simulink model "bldc_lab"  (R2021b)
settings: Solver=ode15s  StartTime=0.0  StopTime=2  FixedStep=0.0000005  MaxStep=0.000001  RelTol=1e-3
undefined symbols (not defined in the file): Ion, Lithium
libraries: spsIGBTDiodeLib x8, slpidlib x2, spsVoltageMeasurementLib x2, spsSeriesRLCBranchLib x2, spsBatteryLib x1, spsCurrentMeasurementLib x1, spsDCVoltageSourceLib x1, spsPermanentMagnetSynchronousMachineLib x1, spsIdealSwitchLib x1, spsPWMGeneratorDCDCLib x1, spspowerguiLib x1
settings Model: Creator=borutzki  LastModifiedBy=borutzki
settings SolverCC: ZeroCrossAlgorithm=Adaptive
settings DebuggingCC: IgnoredZcDiagnostic=none

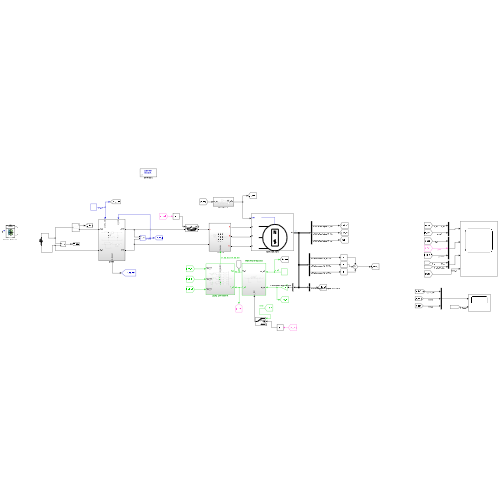
[thumbnail: Simulink's stored preview of the top-level diagram]
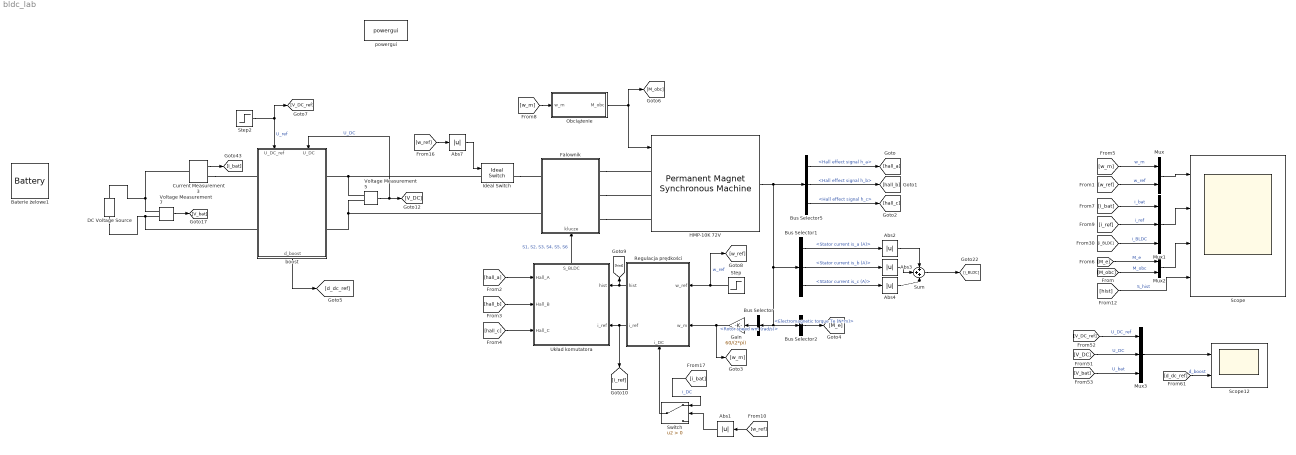
== system bldc_lab ==
  Abs{1..4,7} (5 alike) : Abs
  Baterie żelowe1 : spsBatteryLib/Battery  BatType=Lithium-Ion  ShowTempParam=off  ThermalPreset=no  ShowAgeParam=off  NomV=36  NomQ=5  SOC=100  Batt_Tr=30  PresetModel=on  MaxQ=5  MinV=27  FullV=41.9035  Dis_rate=2.1739  R=0.072  Normal_OP=4.5217  expZone="[38.8939     0.245652]"  current=[6.5 13 32.5]  Units=Time  Tci=20  NomT=20  T2=-30  MaxQ2=4.8  FullV2=7.1  Normal_OP2=5.655  expZone2="[6.58           1]"  Rca=0.6  ti=2000  Dp=0  Neq0=0  Tsim=1e6  Ta1=25  Qeol=5.4*0.9  Reol=0.013333*1.2  Char_age=[2.3478, 3]  Dis_age=[2.3478, 10]  N1=1500  N2=10500  N3=1000  N4=1400  Ta2=45  N5=950
  Bus Selector : BusSelector  OutputSignals=Rotor speed wm (rad/s)
  Bus Selector1 : BusSelector  OutputSignals=Stator current is_a (A),Stator current is_b (A),Stator current is_c (A)
  Bus Selector2 : BusSelector  OutputSignals=Electromagnetic torque Te (N*m)
  Bus Selector5 : BusSelector  OutputSignals=Hall effect signal h_a,Hall effect signal h_b,Hall effect signal h_c
  Current Measurement3 : spsCurrentMeasurementLib/Current Measurement  PhasorSimulation=off  OutputType=Complex  PSBequivalent=0
  DC Voltage Source : spsDCVoltageSourceLib/DC Voltage Source  Amplitude=36  Measurements=None
  Falownik : Subsystem
      settings: PortSchema="{\"entries\":[{\"content\":{\"sides\":[{\"content\":{\"connectorIds\":[\"LConn1\",\"LConn2\"]},\"type\":\"ConnectorPlacement.EquallySpacedRectSide\",\"uuid\":\"21967f67-7ecc-4de4-91fd-b00cf07b6fbf\"},{\"content\":{\"connectorIds\":[\"RConn1\",\"RConn2\",\"RConn3\"],\"side\":\"RIGHT\"},\"type\":\"ConnectorPlacement.EquallySpacedRectSide\",\"uuid\":\"18bc580d-fbaa-4fc1-af99-2ad48ced499f\"},{\"content\":{\"connectorIds\":[],\"side\":\"TOP\"},\"type\":\"ConnectorPlacement.EquallySpacedRectSide\",\"uuid\":\"29f4965a-54f7-4925-8e4b-dbb7ca0827f0\"},{\"content\":{\"connectorIds\":[\"In1\"],\"side\":\"BOTTOM\"},\"type\":\"ConnectorPlacement.EquallySpacedRectSide\",\"uuid\":\"6d9bc2af-b4ca-4c5d-94c1-33ab2980993d\"}]},\"type\":\"ConnectorPlacement.EquallySpacedConnector\",\"uuid\":\"e72db418-b731-4ad1-a158-dfab229f0014\"}],\"packageUris\":[\"http://schema.mathworks.com/mf0/Connector/R2020b\"],\"version\":\"1.0\"}"
  Gain : Gain  Gain=60/(2*pi)
  HMP-10K 72V : spsPermanentMagnetSynchronousMachineLib/Permanent Magnet Synchronous Machine  NbPhases=3  FluxDistribution=Trapezoidal  RotorType=Round  MechanicalLoad=Torque Tm  PresetModel=No  ShowDetailedParameters=on  MeasurementBus=off  Resistance=0.00265  Inductance=5.2e-08  dqInductances=[8.5e-3,8.5e-3]  La=0.000835  MachineConstant=Flux linkage established by magnets (V.s)  Flux=0.0198529  VoltageCst=16.6319  TorqueCst=0.15882  Flat=120  Mechanical=[0.000621417 0 4]  PolePairs=4  InitialConditions=[0,0, 0,0]  InitialConditions5ph=[0 0 0 0 0 0]  RefAngle=90 degrees behind phase A axis (modified Park)  IterativeDiscreteModel=Trapezoidal non iterative  TsBlock=-1  TsPowergui=0
  Ideal Switch : spsIdealSwitchLib/Ideal Switch  Ron=0.001  Lon=0  IC=0  Rs=10e8  Cs=inf  Measurements=on
  Mux : Mux  Inputs=2
  Mux1 : Mux  Inputs=3
  Mux2 : Mux  Inputs=2
  Mux3 : Mux  Inputs=3
  Obciążenie : Subsystem
  Regulacja prędkości : Subsystem
      settings: PortSchema="{\"entries\":[{\"content\":{\"sides\":[{\"content\":{\"connectorIds\":[\"In1\",\"In2\"]},\"type\":\"ConnectorPlacement.EquallySpacedRectSide\",\"uuid\":\"eb00a588-3794-4546-a1d2-9e4e9993d45f\"},{\"content\":{\"connectorIds\":[\"Out1\",\"Out2\"],\"side\":\"RIGHT\"},\"type\":\"ConnectorPlacement.EquallySpacedRectSide\",\"uuid\":\"a8ca2baf-3f9d-4e61-8f3e-3dda34de3f56\"},{\"content\":{\"connectorIds\":[],\"side\":\"TOP\"},\"type\":\"ConnectorPlacement.EquallySpacedRectSide\",\"uuid\":\"d8951c20-e465-4982-8368-20723ce9e6f9\"},{\"content\":{\"connectorIds\":[\"In3\"],\"side\":\"BOTTOM\"},\"type\":\"ConnectorPlacement.EquallySpacedRectSide\",\"uuid\":\"c6264e01-0c9f-421a-afb1-88d153170c6d\"}]},\"type\":\"ConnectorPlacement.EquallySpacedConnector\",\"uuid\":\"1286fe2f-7144-491a-9d4a-5774b4a98f05\"}],\"packageUris\":[\"http://schema.mathworks.com/mf0/Connector/R2020b\"],\"version\":\"1.0\"}"
  Scope : Scope  NumInputPorts=4
  Scope12 : Scope  NumInputPorts=2
  Step : Step  Time=0.5  After=500  SampleTime=0
  Step2 : Step  Time=0.2  After=72  SampleTime=0
  Sum : Sum  Inputs=+++
  Switch : Switch  Criteria=u2 > Threshold
  Układ komutatora : Subsystem
      settings: PortSchema="{\"entries\":[{\"content\":{\"sides\":[{\"content\":{\"connectorIds\":[\"In1\",\"In2\",\"In3\"]},\"type\":\"ConnectorPlacement.EquallySpacedRectSide\",\"uuid\":\"5145dd98-6096-41fa-a175-964c14778fb3\"},{\"content\":{\"connectorIds\":[\"In4\",\"In5\"],\"side\":\"RIGHT\"},\"type\":\"ConnectorPlacement.EquallySpacedRectSide\",\"uuid\":\"5175d556-6ef4-4a11-8093-81f2c4398356\"},{\"content\":{\"connectorIds\":[\"Out1\"],\"side\":\"TOP\"},\"type\":\"ConnectorPlacement.EquallySpacedRectSide\",\"uuid\":\"b6e9d80c-0e29-4a5b-b8c8-415c389c051e\"},{\"content\":{\"connectorIds\":[],\"side\":\"BOTTOM\"},\"type\":\"ConnectorPlacement.EquallySpacedRectSide\",\"uuid\":\"62976cb5-df0e-4349-b1ac-ce6e1718b9a9\"}]},\"type\":\"ConnectorPlacement.EquallySpacedConnector\",\"uuid\":\"8e04dc5d-fea8-4475-a1f4-09d0ee33eb3d\"}],\"packageUris\":[\"http://schema.mathworks.com/mf0/Connector/R2020b\"],\"version\":\"1.0\"}"
  Voltage Measurement5 : spsVoltageMeasurementLib/Voltage Measurement  PhasorSimulation=off  OutputType=Complex  PSBequivalent=0
  Voltage Measurement7 : spsVoltageMeasurementLib/Voltage Measurement  PhasorSimulation=off  OutputType=Complex  PSBequivalent=0
  boost : Subsystem
      settings: PortSchema="{\"entries\":[{\"content\":{\"sides\":[{\"content\":{\"connectorIds\":[\"LConn1\",\"LConn2\"]},\"type\":\"ConnectorPlacement.EquallySpacedRectSide\",\"uuid\":\"4c742702-5063-4be9-90fa-f2ecfe683f39\"},{\"content\":{\"connectorIds\":[\"RConn1\",\"RConn2\"],\"side\":\"RIGHT\"},\"type\":\"ConnectorPlacement.EquallySpacedRectSide\",\"uuid\":\"6758a030-dee0-40f5-ab65-dbe6d9640e0b\"},{\"content\":{\"connectorIds\":[\"In1\",\"In2\"],\"side\":\"TOP\"},\"type\":\"ConnectorPlacement.EquallySpacedRectSide\",\"uuid\":\"71135b2c-1a2a-4dc9-8a7c-02ce7c2ac3cd\"},{\"content\":{\"connectorIds\":[\"Out1\"],\"side\":\"BOTTOM\"},\"type\":\"ConnectorPlacement.EquallySpacedRectSide\",\"uuid\":\"cd62799b-22c9-45d9-9a7c-0387e77ecd9b\"}]},\"type\":\"ConnectorPlacement.EquallySpacedConnector\",\"uuid\":\"113fdbd2-88dc-4715-bf53-b53f7b5d75de\"}],\"packageUris\":[\"http://schema.mathworks.com/mf0/Connector/R2020b\"],\"version\":\"1.0\"}"
  powergui : spspowerguiLib/powergui  Priority=1  SimulationMode=Discrete  SampleTime=0.000005  frequency=60  Iterations=50  frequencyindice=0  Pbase=100e6  ErrMax=1e-4  UnitsV=kV  UnitsW=MW  buscounter=0  FunctionMessages=off  echomessages=off  EnableUseOfTLC=off  CurrentSourceSwitches=off  DisableSnubberDevices=off  DisableRonSwitches=off  DisableVfSwitches=off  DisplayEquations=off  AutomaticDiscreteSolvers=on  SolverType=Tustin/Backward Euler (TBE)  Interpol=off  ExternalGateDelay=off  methode=off  Ts=100  x0status=blocks  SPID=on  SwTol=0  HookPort=off  NonlinearTolerance=1e-4  nMaxIteration=100  ContinueOnMaxIteration=off  RestoreLinks=warning  ResistiveCurrentMeasurement=off  Frange=[0:2:500]  Ylog=off  Xlog=on  ShowGrid=off  save=off  variable=ZData  structure=0  ZoomFFT=off  StartTime=0.0  cycles=1  DisplayStyle=1  fundamental=60  FreqAxis=off  MaxFrequency=1000  frequencyindicesteady=1  RmsSteady=1  display=off
  wires:
  Bus Selector5/1 -> [hall_a]  "<Hall effect signal h_a>"
  Bus Selector5/2 -> [hall_b]  "<Hall effect signal h_b>"
  Bus Selector5/3 -> [hall_c]  "<Hall effect signal h_c>"
  [i_bat] -> Mux1/1  "i_bat"
  Voltage Measurement5/1 -> boost/2(U_DC), [V_DC]  "U_DC"
  Voltage Measurement7/1 -> [V_bat]
  Current Measurement3/1 -> [i_bat]
  [d_dc_ref] -> Scope12/2  "d_boost"
  [V_bat] -> Mux3/3  "U_bat"
  Mux3/1 -> Scope12/1
  [V_DC_ref] -> Mux3/1  "U_DC_ref"
  [V_DC] -> Mux3/2  "U_DC"
  [w_m] -> Mux/1  "w_m"
  [w_ref] -> Mux/2  "w_ref"
  Mux/1 -> Scope/1
  [i_ref] -> Mux1/2  "i_ref"
  Mux1/1 -> Scope/2
  [hist] -> Scope/4  "S_hist"
  Bus Selector1/3 -> Abs4/1  "<Stator current is_c (A)>"
  Bus Selector1/2 -> Abs3/1  "<Stator current is_b (A)>"
  Bus Selector1/1 -> Abs2/1  "<Stator current is_a (A)>"
  Abs2/1 -> Sum/1
  Abs3/1 -> Sum/2
  Abs4/1 -> Sum/3
  Sum/1 -> [i_BLDC]
  [i_BLDC] -> Mux1/3  "i_BLDC"
  [w_ref] -> Abs7/1
  Abs7/1 -> Ideal Switch/1
  Step2/1 -> boost/1(U_DC_ref), [V_DC_ref]  "U_ref"
  boost/1(d_boost) -> [d_dc_ref]
  [w_m] -> Obciążenie/1(w_m)
  [hall_a] -> Układ komutatora/1(Hall_A)
  [hall_b] -> Układ komutatora/2(Hall_B)
  [hall_c] -> Układ komutatora/3(Hall_C)
  Układ komutatora/1(S_BLDC) -> Falownik/1(klucze)  "S1, S2, S3, S4, S5, S6"
  Regulacja prędkości/1(hist) -> Układ komutatora/4(hist), [hist]
  Regulacja prędkości/2(i_ref) -> [i_ref], Układ komutatora/5(i_ref)
  Step/1 -> [w_ref], Regulacja prędkości/1(w_ref)  "w_ref"
  HMP-10K 72V/1 -> Bus Selector2/1, Bus Selector/1, Bus Selector1/1, Bus Selector5/1
  Bus Selector/1 -> Gain/1  "<Rotor speed wm (rad/s)>"
  Gain/1 -> [w_m], Regulacja prędkości/2(w_m)
  [i_bat] -> Switch/1  "i_DC"
  Obciążenie/1(M_obc) -> [M_obc], HMP-10K 72V/1
  Bus Selector2/1 -> [M_e]  "<Electromagnetic torque Te (N*m)>"
  [M_e] -> Mux2/1  "M_e"
  [M_obc] -> Mux2/2  "M_obc"
  Mux2/1 -> Scope/3
  [w_ref] -> Abs1/1
  Abs1/1 -> Switch/2
  Switch/1 -> Regulacja prędkości/3(i_DC)
  connections:
  Falownik/RConn1 -- HMP-10K 72V/LConn1
  Falownik/RConn2 -- HMP-10K 72V/LConn2
  Falownik/RConn3 -- HMP-10K 72V/LConn3
  Falownik/LConn2 -- boost/RConn2 -- Voltage Measurement5/LConn2
  Current Measurement3/LConn1 -- DC Voltage Source/RConn1 -- Voltage Measurement7/LConn1
  Voltage Measurement5/LConn1 -- boost/RConn1 -- Ideal Switch/LConn1
  Ideal Switch/RConn1 -- Falownik/LConn1
  Voltage Measurement7/LConn2 -- DC Voltage Source/LConn1 -- boost/LConn2
  Current Measurement3/RConn1 -- boost/LConn1

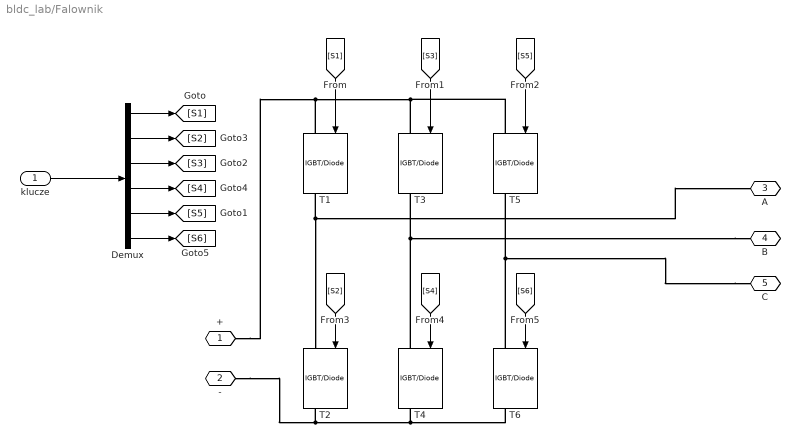
== system bldc_lab/Falownik ==
  klucze : Inport
  Demux : Demux  Outputs=6
  T{1..6} (6 alike) : spsIGBTDiodeLib/IGBT//Diode  Ron=1e-3  Rs=1e5  Cs=inf  Measurements=on
  + : PMIOPort  Side=Left
  - : PMIOPort  Port=2  Side=Left
  A : PMIOPort  Port=3  Side=Right
  B : PMIOPort  Port=4  Side=Right
  C : PMIOPort  Port=5  Side=Right
  wires:
  [S4] -> T4/1
  [S6] -> T6/1
  [S2] -> T2/1
  [S5] -> T5/1
  [S3] -> T3/1
  klucze/1 -> Demux/1
  Demux/1 -> [S1]
  Demux/2 -> [S2]
  Demux/3 -> [S3]
  Demux/4 -> [S4]
  Demux/5 -> [S5]
  Demux/6 -> [S6]
  [S1] -> T1/1
  connections:
  -/RConn1 -- T6/RConn1 -- T4/RConn1 -- T2/RConn1
  T1/RConn1 -- T2/LConn1 -- A/RConn1
  B/RConn1 -- T4/LConn1 -- T3/RConn1
  +/RConn1 -- T1/LConn1 -- T5/LConn1 -- T3/LConn1
  C/RConn1 -- T6/LConn1 -- T5/RConn1

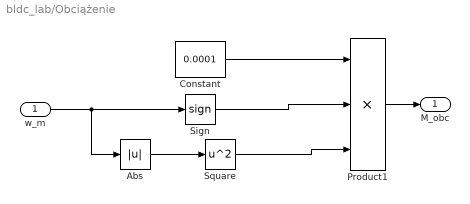
== system bldc_lab/Obciążenie ==
  w_m : Inport
  Abs : Abs
  Constant : Constant  Value=0.0001
  Product1 : Product  Inputs=3
  Sign : Signum
  Square : Math  Operator=square  SaturateOnIntegerOverflow=on
  M_obc : Outport
  wires:
  Product1/1 -> M_obc/1
  Square/1 -> Product1/3
  Abs/1 -> Square/1
  Constant/1 -> Product1/1
  w_m/1 -> Abs/1, Sign/1
  Sign/1 -> Product1/2

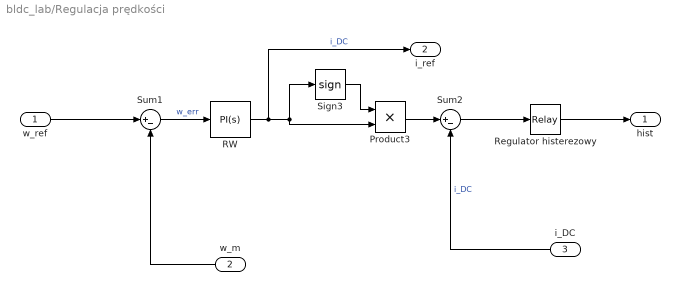
== system bldc_lab/Regulacja prędkości ==
  w_ref : Inport
  w_m : Inport  Port=2
  i_DC : Inport  Port=3
  Product3 : Product
  RW : slpidlib/PID Controller  Controller=PI  Form=Parallel  TimeDomain=Continuous-time  UseExternalTs=off  SampleTime=-1  IntegratorMethod=Forward Euler  FilterMethod=Forward Euler  ControllerParametersSource=internal  P=2  I=10  D=0  UseFilter=on  N=100  TunerSelectOption=Transfer Function Based (PID Tuner App)  InitialConditionSource=internal  InitialConditionForIntegrator=0  InitialConditionForFilter=0  DifferentiatorICPrevScaledInput=0  ExternalReset=none  TrackingMode=off  Kt=1  LimitOutput=on  SatLimitsSource=internal  UpperSaturationLimit=200  LowerSaturationLimit=-200  LinearizeAsGain=on  AntiWindupMode=clamping  Kb=1  POutMin=[]  POutMax=[]  IOutMin=[]  IOutMax=[]  DOutMin=[]  DOutMax=[]  NOutMin=[]  NOutMax=[]  SumOutMin=[]  SumOutMax=[]  SaturationOutMin=[]  SaturationOutMax=[]  PParamMin=[]  PParamMax=[]  IParamMin=[]  IParamMax=[]  DParamMin=[]  DParamMax=[]  NParamMin=[]  NParamMax=[]  KbParamMin=[]  KbParamMax=[]  KtParamMin=[]  KtParamMax=[]  KbOutMin=[]  KbOutMax=[]  KtOutMin=[]  KtOutMax=[]  IntegratorOutMin=[]  IntegratorOutMax=[]  FilterOutMin=[]  FilterOutMax=[]  SumI1OutMin=[]  SumI1OutMax=[]  SumI2OutMin=[]  SumI2OutMax=[]  SumI3OutMin=[]  SumI3OutMax=[]  SumI4OutMin=[]  SumI4OutMax=[]  SumDOutMin=[]  SumDOutMax=[]  DifferentiatorOutMin=[]  DifferentiatorOutMax=[]  FilterDiffOutCoefMin=[]  FilterDiffOutCoefMax=[]  ReciprocalOutMin=[]  ReciprocalOutMax=[]  SumDenOutMin=[]  SumDenOutMax=[]  SumNumOutMin=[]  SumNumOutMax=[]  DivideOutMin=[]  DivideOutMax=[]  UdiffTsProdOutMin=[]  UdiffTsProdOutMax=[]  NTsProdOutMin=[]  NTsProdOutMax=[]  UintegralTsProdOutMin=[]  UintegralTsProdOutMax=[]  UngainTsProdOutMin=[]  UngainTsProdOutMax=[]  IntegratorContinuousStateAttributes=''  IntegratorStateMustResolveToSignalObject=off  IntegratorRTWStateStorageClass=Auto  FilterContinuousStateAttributes=''  FilterStateMustResolveToSignalObject=off  FilterRTWStateStorageClass=Auto  ParallelPVariant=InternalParameters  IdealPVariant=Disabled  IVariant=InternalParameters  DVariant=Disabled  IntegratorVariant=Continuous  SatVariant=Enabled  AWVariant=ContClampingParallel  PCopyVariant=Disabled  TRVariant=Disabled  FdbkBlocksVariant=Forward  IdealPFdbkVariant=Disabled  SatFdbkVariant=Disabled  DerivativeFilterVariant=Disabled  NVariant=Disabled  NCopyVariant=Disabled_SignalSpec  FilterICVariant=Disabled  IntegratorICVariant=InternalICs  ExternalResetVariant=Disabled  TRSumVariant=Passthrough  SumFdbkVariant=Disabled  SumVariant=Sum_PI  TsampFilterVariant=InternalTs  TsampNgainVariant=Passthrough  TsampIntegralVariant=Passthrough  ExternalSaturationOutDataTypeStr=Inherit: Same as second input
  Regulator histerezowy : Relay  OnSwitchValue=0.0001  OffSwitchValue=-0.0001
  Sign3 : Signum
  Sum1 : Sum  Inputs=|+-
  Sum2 : Sum  Inputs=|+-
  hist : Outport
  i_ref : Outport  Port=2
  wires:
  Regulator histerezowy/1 -> hist/1
  i_DC/1 -> Sum2/2  "i_DC"
  Product3/1 -> Sum2/1
  Sign3/1 -> Product3/1
  RW/1 -> i_ref/1, Product3/2, Sign3/1  "i_DC"
  w_m/1 -> Sum1/2
  Sum2/1 -> Regulator histerezowy/1
  w_ref/1 -> Sum1/1
  Sum1/1 -> RW/1  "w_err"

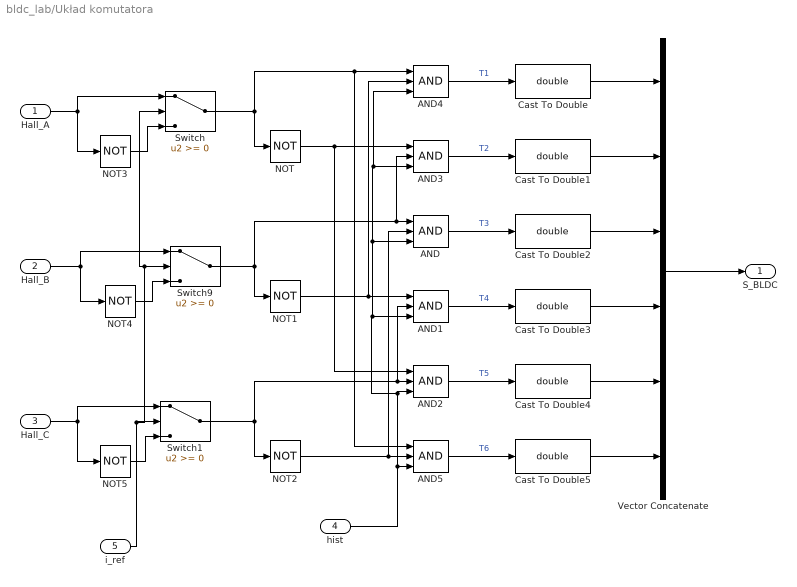
== system bldc_lab/Układ komutatora ==
  Hall_A : Inport
  Hall_B : Inport  Port=2
  Hall_C : Inport  Port=3
  hist : Inport  Port=4
  i_ref : Inport  Port=5
  AND{,1..5} (6 alike) : Logic  Inputs=3  IconShape=distinctive  AllPortsSameDT=off
  Cast To Double{,1..5} (6 alike) : DataTypeConversion  OutDataTypeStr=double
  NOT{,1..5} (6 alike) : Logic  Operator=NOT  IconShape=distinctive  AllPortsSameDT=off  OutDataTypeStr=boolean
  Switch : Switch
  Switch1 : Switch
  Switch9 : Switch
  Vector Concatenate : Concatenate  NumInputs=6
  S_BLDC : Outport
  wires:
  NOT/1 -> AND3/1, AND2/1
  Hall_C/1 -> Switch1/1, NOT5/1
  Cast To Double1/1 -> Vector Concatenate/2
  i_ref/1 -> Switch/2, Switch9/2, Switch1/2
  Cast To Double/1 -> Vector Concatenate/1
  Switch/1 -> NOT/1, AND5/1, AND4/1
  hist/1 -> AND4/3, AND3/3, AND/3, AND1/3, AND2/3, AND5/3
  Hall_B/1 -> Switch9/1, NOT4/1
  NOT3/1 -> Switch/3
  Vector Concatenate/1 -> S_BLDC/1
  AND4/1 -> Cast To Double/1  "T1"
  Hall_A/1 -> Switch/1, NOT3/1
  NOT5/1 -> Switch1/3
  AND3/1 -> Cast To Double1/1  "T2"
  NOT4/1 -> Switch9/3
  Cast To Double5/1 -> Vector Concatenate/6
  AND2/1 -> Cast To Double4/1  "T5"
  NOT1/1 -> AND1/1, AND4/2
  Switch1/1 -> NOT2/1, AND1/2, AND2/2
  NOT2/1 -> AND/2, AND5/2
  Cast To Double4/1 -> Vector Concatenate/5
  AND1/1 -> Cast To Double3/1  "T4"
  Cast To Double2/1 -> Vector Concatenate/3
  AND5/1 -> Cast To Double5/1  "T6"
  AND/1 -> Cast To Double2/1  "T3"
  Switch9/1 -> NOT1/1, AND3/2, AND/1
  Cast To Double3/1 -> Vector Concatenate/4

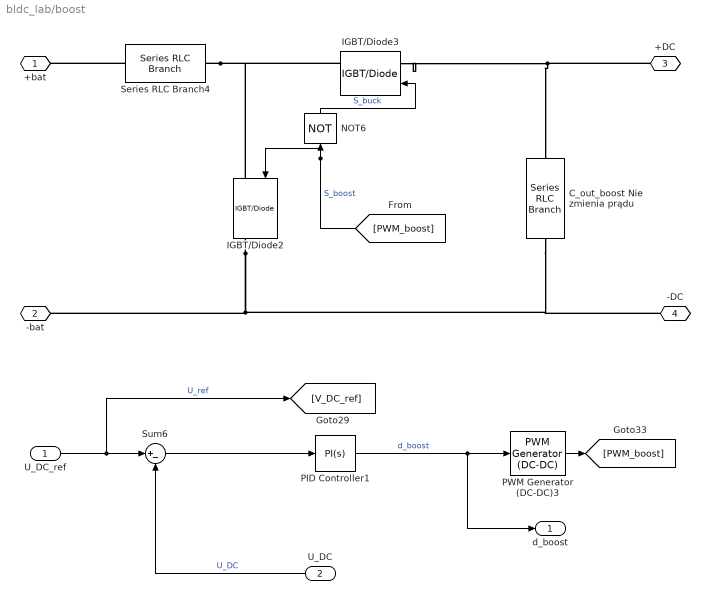
== system bldc_lab/boost ==
  U_DC_ref : Inport
  U_DC : Inport  Port=2
  C_out_boost Nie zmienia prądu : spsSeriesRLCBranchLib/Series RLC Branch  LConnTagsString=__new0  RConnTagsString=__new0  BranchType=C  Resistance=0.005  Inductance=1e-3  SetiL0=off  InitialCurrent=0  Capacitance=0.06  Setx0=off  InitialVoltage=52.2  Measurements=None
  IGBT/Diode2 : spsIGBTDiodeLib/IGBT//Diode  Ron=1e-3  Rs=1e5  Cs=inf  Measurements=on
  IGBT/Diode3 : spsIGBTDiodeLib/IGBT//Diode  Ron=1e-3  Rs=1e5  Cs=inf  Measurements=on
  NOT6 : Logic  Operator=NOT  IconShape=distinctive  AllPortsSameDT=off  OutDataTypeStr=boolean
  PID Controller1 : slpidlib/PID Controller  Controller=PI  Form=Parallel  TimeDomain=Continuous-time  UseExternalTs=off  SampleTime=-1  IntegratorMethod=Forward Euler  FilterMethod=Forward Euler  ControllerParametersSource=internal  P=0.05  I=0.05  D=0  UseFilter=on  N=100  TunerSelectOption=Transfer Function Based (PID Tuner App)  InitialConditionSource=internal  InitialConditionForIntegrator=0  InitialConditionForFilter=0  DifferentiatorICPrevScaledInput=0  ExternalReset=none  TrackingMode=off  Kt=1  LimitOutput=on  SatLimitsSource=internal  UpperSaturationLimit=0.9  LowerSaturationLimit=0  LinearizeAsGain=on  AntiWindupMode=clamping  Kb=1  POutMin=[]  POutMax=[]  IOutMin=[]  IOutMax=[]  DOutMin=[]  DOutMax=[]  NOutMin=[]  NOutMax=[]  SumOutMin=[]  SumOutMax=[]  SaturationOutMin=[]  SaturationOutMax=[]  PParamMin=[]  PParamMax=[]  IParamMin=[]  IParamMax=[]  DParamMin=[]  DParamMax=[]  NParamMin=[]  NParamMax=[]  KbParamMin=[]  KbParamMax=[]  KtParamMin=[]  KtParamMax=[]  KbOutMin=[]  KbOutMax=[]  KtOutMin=[]  KtOutMax=[]  IntegratorOutMin=[]  IntegratorOutMax=[]  FilterOutMin=[]  FilterOutMax=[]  SumI1OutMin=[]  SumI1OutMax=[]  SumI2OutMin=[]  SumI2OutMax=[]  SumI3OutMin=[]  SumI3OutMax=[]  SumI4OutMin=[]  SumI4OutMax=[]  SumDOutMin=[]  SumDOutMax=[]  DifferentiatorOutMin=[]  DifferentiatorOutMax=[]  FilterDiffOutCoefMin=[]  FilterDiffOutCoefMax=[]  ReciprocalOutMin=[]  ReciprocalOutMax=[]  SumDenOutMin=[]  SumDenOutMax=[]  SumNumOutMin=[]  SumNumOutMax=[]  DivideOutMin=[]  DivideOutMax=[]  UdiffTsProdOutMin=[]  UdiffTsProdOutMax=[]  NTsProdOutMin=[]  NTsProdOutMax=[]  UintegralTsProdOutMin=[]  UintegralTsProdOutMax=[]  UngainTsProdOutMin=[]  UngainTsProdOutMax=[]  IntegratorContinuousStateAttributes=''  IntegratorStateMustResolveToSignalObject=off  IntegratorRTWStateStorageClass=Auto  FilterContinuousStateAttributes=''  FilterStateMustResolveToSignalObject=off  FilterRTWStateStorageClass=Auto  ParallelPVariant=InternalParameters  IdealPVariant=Disabled  IVariant=InternalParameters  DVariant=Disabled  IntegratorVariant=Continuous  SatVariant=Enabled  AWVariant=ContClampingParallel  PCopyVariant=Disabled  TRVariant=Disabled  FdbkBlocksVariant=Forward  IdealPFdbkVariant=Disabled  SatFdbkVariant=Disabled  DerivativeFilterVariant=Disabled  NVariant=Disabled  NCopyVariant=Disabled_SignalSpec  FilterICVariant=Disabled  IntegratorICVariant=InternalICs  ExternalResetVariant=Disabled  TRSumVariant=Passthrough  SumFdbkVariant=Disabled  SumVariant=Sum_PI  TsampFilterVariant=InternalTs  TsampNgainVariant=Passthrough  TsampIntegralVariant=Passthrough  ExternalSaturationOutDataTypeStr=Inherit: Same as second input
  PWM Generator (DC-DC)3 : spsPWMGeneratorDCDCLib/PWM Generator (DC-DC)  Fsw=10000  Ts=0
  Series RLC Branch4 : spsSeriesRLCBranchLib/Series RLC Branch  LConnTagsString=__new0  RConnTagsString=__new0  BranchType=L  Resistance=0.0001  Inductance=0.001  SetiL0=off  InitialCurrent=0  Capacitance=1e-6  Setx0=off  InitialVoltage=0  Measurements=None
  Sum6 : Sum  Inputs=|+-
  +bat : PMIOPort  Side=Left
  -bat : PMIOPort  Port=2  Side=Left
  +DC : PMIOPort  Port=3  Side=Right
  -DC : PMIOPort  Port=4  Side=Right
  d_boost : Outport
  wires:
  NOT6/1 -> IGBT/Diode3/1  "S_buck"
  [PWM_boost] -> IGBT/Diode2/1, NOT6/1  "S_boost"
  U_DC_ref/1 -> [V_DC_ref], Sum6/1  "U_ref"
  Sum6/1 -> PID Controller1/1
  PID Controller1/1 -> d_boost/1, PWM Generator (DC-DC)3/1  "d_boost"
  PWM Generator (DC-DC)3/1 -> [PWM_boost]
  U_DC/1 -> Sum6/2  "U_DC"
  connections:
  IGBT/Diode2/RConn1 -- -bat/RConn1 -- -DC/RConn1 -- C_out_boost Nie zmienia prądu/RConn1
  Series RLC Branch4/RConn1 -- IGBT/Diode3/RConn1 -- IGBT/Diode2/LConn1
  IGBT/Diode3/LConn1 -- +DC/RConn1 -- C_out_boost Nie zmienia prądu/LConn1
  Series RLC Branch4/LConn1 -- +bat/RConn1
